simulink model "Problem3"  (R2020b)
settings: Solver=VariableStepAuto  StartTime=0.0  StopTime=10.0  RelTol=1e-3
settings Model: Creator=ASUS  LastModifiedBy=ASUS

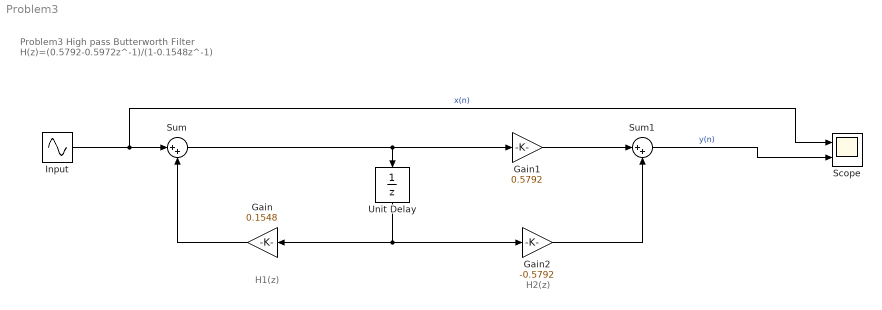
== system Problem3 ==
  note: Problem3
      | High pass Butterworth Filter
      | H(z)=(0.5792-0.5972z^-1)/(1-0.1548z^-1)
  note: H2(z)
  note: H1(z)
  Gain : Gain  Gain=0.1548
  Gain1 : Gain  Gain=0.5792
  Gain2 : Gain  Gain=-0.5792
  Input : Sin  Frequency=100*2*pi  SampleTime=0
  Scope : Scope  NumInputPorts=2
  Sum : Sum  Inputs=|++
  Sum1 : Sum  Inputs=|++
  Unit Delay : UnitDelay  SampleTime=-1  HasFrameUpgradeWarning=on
  wires:
  Gain1/1 -> Sum1/1
  Sum/1 -> Gain1/1, Unit Delay/1
  Unit Delay/1 -> Gain2/1, Gain/1
  Gain2/1 -> Sum1/2
  Gain/1 -> Sum/2
  Input/1 -> Scope/1, Sum/1  "x(n)"
  Sum1/1 -> Scope/2  "y(n)"
